simulink model "Punto6_4"  (R2017a)
settings: Solver=VariableStepAuto  StartTime=0.0  StopTime=10.0  RelTol=1e-3
values from neighbouring files (symbols this model uses):
  dena = [1 4]    [Punto_6_4.m]    (also in Punto_6_5.m = [1 -0.9231])
  denb = [1 8 25]    [Punto_6_4.m]    (also in Punto_6_5.m = [1 -1.847 0.8521])
  denc = [1 8 29 52]    [Punto_6_4.m]    (also in Punto_6_5.m = [1 -36 0.168 -0.02556])
  numa = 2    [Punto_6_4.m]    (also in Punto_6_5.m = 0.06727)
  numb = 50    [Punto_6_4.m]    (also in Punto_6_5.m = [0.01847 0.001847])
  numc = 26    [Punto_6_4.m]    (also in Punto_6_5.m = [0.1411 0.2112 0.0224])
undefined symbols (not defined in the file or in its folder): aa, ab, ac, ba, bb, bc, ca, cb, cc
settings Model: Creator=franj  LastModifiedBy=franj

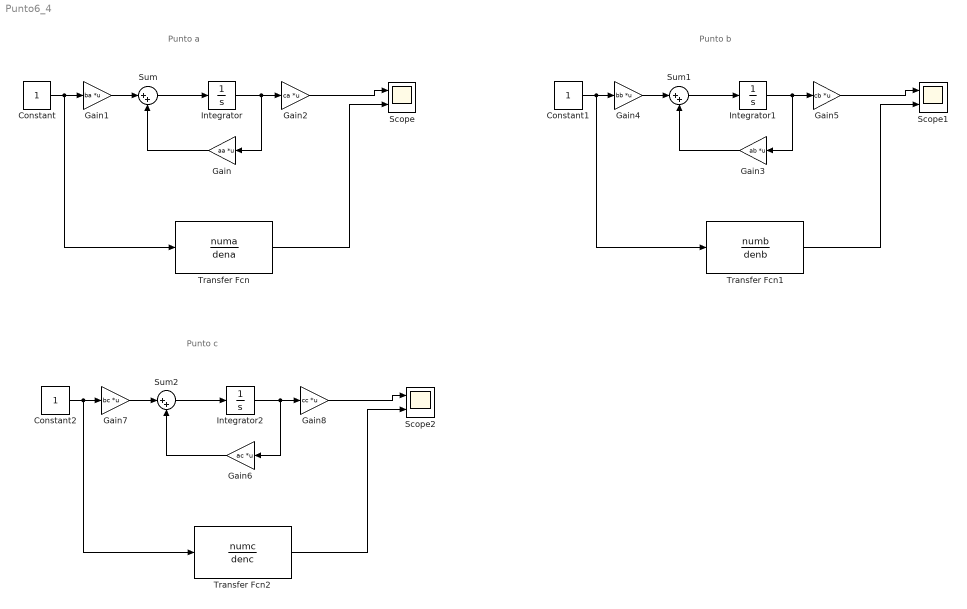
== system Punto6_4 ==
  note: Punto a
  note: Punto b
  note: Punto c
  Constant : Constant
  Constant1 : Constant
  Constant2 : Constant
  Gain : Gain  Gain=aa  Multiplication=Matrix(K*u)
  Gain1 : Gain  Gain=ba  Multiplication=Matrix(K*u)
  Gain2 : Gain  Gain=ca  Multiplication=Matrix(K*u)
  Gain3 : Gain  Gain=ab  Multiplication=Matrix(K*u)
  Gain4 : Gain  Gain=bb  Multiplication=Matrix(K*u)
  Gain5 : Gain  Gain=cb  Multiplication=Matrix(K*u)
  Gain6 : Gain  Gain=ac  Multiplication=Matrix(K*u)
  Gain7 : Gain  Gain=bc  Multiplication=Matrix(K*u)
  Gain8 : Gain  Gain=cc  Multiplication=Matrix(K*u)
  Integrator : Integrator
  Integrator1 : Integrator
  Integrator2 : Integrator
  Scope : Scope  NumInputPorts=2
  Scope1 : Scope  NumInputPorts=2
  Scope2 : Scope  NumInputPorts=2
  Sum : Sum  Inputs=|++
  Sum1 : Sum  Inputs=|++
  Sum2 : Sum  Inputs=|++
  Transfer Fcn : TransferFcn  Numerator=numa  Denominator=dena
  Transfer Fcn1 : TransferFcn  Numerator=numb  Denominator=denb
  Transfer Fcn2 : TransferFcn  Numerator=numc  Denominator=denc
  wires:
  Constant/1 -> Transfer Fcn/1, Gain1/1
  Gain1/1 -> Sum/1
  Sum/1 -> Integrator/1
  Integrator/1 -> Gain/1, Gain2/1
  Gain/1 -> Sum/2
  Gain2/1 -> Scope/1
  Transfer Fcn/1 -> Scope/2
  Integrator1/1 -> Gain3/1, Gain5/1
  Transfer Fcn1/1 -> Scope1/2
  Gain3/1 -> Sum1/2
  Gain4/1 -> Sum1/1
  Constant1/1 -> Transfer Fcn1/1, Gain4/1
  Sum1/1 -> Integrator1/1
  Gain5/1 -> Scope1/1
  Integrator2/1 -> Gain6/1, Gain8/1
  Transfer Fcn2/1 -> Scope2/2
  Gain6/1 -> Sum2/2
  Gain7/1 -> Sum2/1
  Constant2/1 -> Transfer Fcn2/1, Gain7/1
  Sum2/1 -> Integrator2/1
  Gain8/1 -> Scope2/1
